simulink model "Practica_4"  (R2020b)
settings: Solver=VariableStepAuto  StartTime=0.0  StopTime=inf  RelTol=1e-3
model workspace (MAT data in the model file):
  alpha = Simulink.Parameter
  alpha.Value = 0.04
  alpha.DataType = 'auto'
  alpha.Dimensions = [1 1]
  dt = Simulink.Parameter
  dt.Value = 0.01
  dt.DataType = 'auto'
  dt.Dimensions = [1 1]
undefined symbols (not defined in the file or in its folder): serial
libraries: instrumentlib x2
settings Model: EnablePacing=on  Creator=eber_  LastModifiedBy=eber_

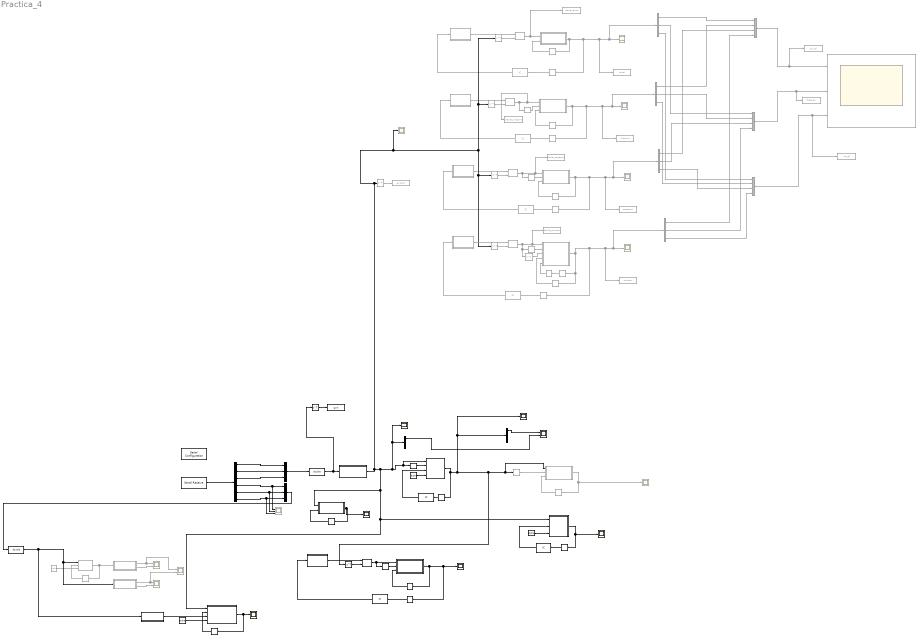
== system Practica_4 ==
  #nofilter : Scope  Commented=on  NumInputPorts=2
  #nofilter1 : Scope  Commented=on  NumInputPorts=2
  Chart : Stateflow chart  TreatAsAtomicUnit=on
  Data Type Conversion : DataTypeConversion  OutDataTypeStr=double
  Data Type Conversion2 : DataTypeConversion  OutDataTypeStr=double
  Delay : Delay  Commented=on
  Demux{,1..3} (4 alike) : Demux  Commented=on  Outputs=3
  Demux4 : Demux  Outputs=6
  Demux6 : Demux  Outputs=3
  Demux7 : Demux  Outputs=3
  Eul Angles{,2..4} (4 alike) : Scope  Commented=on
  Eul Angles1 : Scope
  Euler : MATLAB Function  Commented=on  TreatAsAtomicUnit=on
  Euler1 : MATLAB Function  TreatAsAtomicUnit=on
  Gyro1 : Scope  Commented=on
  IC{,2..4} (4 alike) : InitialCondition  Commented=on  Value=[0; 0; 0]
  IC1 : InitialCondition  Value=[0, 0, 0]
  IC5 : InitialCondition  Value=[0, 0, 0]
  IC6 : InitialCondition  Value=[0; 0; 0]
  MATLAB Function : MATLAB Function  Commented=on  TreatAsAtomicUnit=on
  MATLAB Function1 : MATLAB Function  Commented=on  TreatAsAtomicUnit=on
  MATLAB Function2 : MATLAB Function  Commented=on  TreatAsAtomicUnit=on
  MATLAB Function3 : MATLAB Function  TreatAsAtomicUnit=on
  MATLAB Function4 : MATLAB Function  TreatAsAtomicUnit=on
  MATLAB Function5 : MATLAB Function  TreatAsAtomicUnit=on
  MATLAB Function6 : MATLAB Function  TreatAsAtomicUnit=on
  Matrix Multiply{,1..3} (4 alike) : Product  Commented=on  Multiplication=Matrix(*)
  Matrix Multiply4 : Product  Multiplication=Matrix(*)
  Memory{,1..8,10..11,15} (12 alike) : Memory  Commented=on
  Memory12 : Memory  Commented=on  InheritSampleTime=on
  Memory13 : Memory  Commented=on  InheritSampleTime=on
  Memory14 : Memory  Commented=on  InitialCondition=[0, 0, 0]
  Memory{16,18..23} (7 alike) : Memory
  Memory17 : Memory  InitialCondition=[0, 0, 0]
  Memory9 : Memory  Commented=on  InheritSampleTime=on
  Midpoint : MATLAB Function  Commented=on  TreatAsAtomicUnit=on
  Mux : Mux  Commented=on
  Mux1 : Mux  Commented=on
  Mux2 : Mux  Commented=on
  Mux3 : Mux  Inputs=3
  Mux4 : Mux  Inputs=3
  Scope : Scope  Commented=on  NumInputPorts=3
  Scope1 : Scope  Commented=on
  Scope2 : Scope  Commented=on  NumInputPorts=3
  Scope{3..4,6..8} (5 alike) : Scope
  Scope5 : Scope  NumInputPorts=2
  Serial Configuration : instrumentlib/Serial Configuration  Priority=-200000  ComPortMenu=<Please select a port...>  ComPort=COM3  ObjConstructor=serial('COM3');  BaudRate=115200  DataBits=8  Parity=none  StopBits=1  FlowControl=none  Timeout=10  ByteOrder=LittleEndian
  Serial Receive : instrumentlib/Serial Receive  ComPortMenu=<Please select a port...>  ComPort=COM3  ObjConstructor=serial('COM3');  Terminator=<none>  DataSize="[1  6]"  DataType=single  EnableBlockingMode=on  ActionDataUnavailable=Output last received value  CustomValue=0  SampleTime=0.02
  Simpson : MATLAB Function  Commented=on  TreatAsAtomicUnit=on
  To Workspace1 : ToWorkspace  Commented=on  VariableName=euler  SaveFormat=Structure With Time  SampleTime=-1
  To Workspace10 : ToWorkspace  Commented=on  VariableName=deuler_simpson  SaveFormat=Structure With Time  SampleTime=-1
  To Workspace11 : ToWorkspace  Commented=on  VariableName=psi_all  SaveFormat=Structure With Time  SampleTime=-1
  To Workspace12 : ToWorkspace  Commented=on  VariableName=theta_all  SaveFormat=Structure With Time  SampleTime=-1
  To Workspace13 : ToWorkspace  Commented=on  VariableName=phi_all  SaveFormat=Structure With Time  SampleTime=-1
  To Workspace2 : ToWorkspace  VariableName=gyro  SaveFormat=Structure With Time  SampleTime=-1
  To Workspace3 : ToWorkspace  Commented=on  VariableName=gyrocorr  SaveFormat=Structure With Time  SampleTime=-1
  To Workspace4 : ToWorkspace  Commented=on  VariableName=midpoint  SaveFormat=Structure With Time  SampleTime=-1
  To Workspace5 : ToWorkspace  Commented=on  VariableName=trapezoid  SaveFormat=Structure With Time  SampleTime=-1
  To Workspace6 : ToWorkspace  Commented=on  VariableName=simpson  SaveFormat=Structure With Time  SampleTime=-1
  To Workspace7 : ToWorkspace  Commented=on  VariableName=deuler_euler  SaveFormat=Structure With Time  SampleTime=-1
  To Workspace8 : ToWorkspace  Commented=on  VariableName=deuler_midpoint  SaveFormat=Structure With Time  SampleTime=-1
  To Workspace9 : ToWorkspace  Commented=on  VariableName=deuler_trapezoid  SaveFormat=Structure With Time  SampleTime=-1
  Transformation Matrix : MATLAB Function  Commented=on  TreatAsAtomicUnit=on
  Transformation Matrix1 : MATLAB Function  Commented=on  TreatAsAtomicUnit=on
  Transformation Matrix2 : MATLAB Function  Commented=on  TreatAsAtomicUnit=on
  Transformation Matrix3 : MATLAB Function  Commented=on  TreatAsAtomicUnit=on
  Transformation Matrix4 : MATLAB Function  TreatAsAtomicUnit=on
  Transpose{,1..3,5} (5 alike) : Math  Commented=on  Operator=transpose  SaturateOnIntegerOverflow=on
  Transpose4 : Math  Operator=transpose  SaturateOnIntegerOverflow=on
  Transpose6 : Math  Operator=transpose  SaturateOnIntegerOverflow=on
  Trapezoid : MATLAB Function  Commented=on  TreatAsAtomicUnit=on
  Trapezoid1 : MATLAB Function  Commented=on  TreatAsAtomicUnit=on
  Trapezoid2 : MATLAB Function  TreatAsAtomicUnit=on
  alpha : Constant  Commented=on  Value=alpha
  alpha1 : Constant  Value=alpha
  alpha2 : Constant  Value=alpha
  alpha3 : Constant  Value=alpha
  filtered : Scope  Commented=on  NumInputPorts=2
  wires:
  Data Type Conversion/1 -> Transpose4/1, Chart/1(gyroIn)
  Euler/1(Euler_out) -> Memory/1, Memory1/1, To Workspace1/1, Eul Angles/1, Demux3/1
  IC/1 -> Transformation Matrix/1(Phi)
  Memory1/1 -> IC/1
  Memory/1 -> Euler/2(Euler)
  Transformation Matrix/1(H) -> Matrix Multiply/1
  Transpose/1 -> Matrix Multiply/2
  Matrix Multiply/1 -> To Workspace7/1, Euler/1(Euler_dot)
  Matrix Multiply1/1 -> Memory4/1, To Workspace8/1, Midpoint/1(Euler_dot)
  Transpose1/1 -> Matrix Multiply1/2
  Transformation Matrix1/1(H) -> Matrix Multiply1/1
  Memory3/1 -> Midpoint/3(Euler)
  Memory5/1 -> IC2/1
  IC2/1 -> Transformation Matrix1/1(Phi)
  Midpoint/1(Euler_out) -> Demux2/1, Eul Angles2/1, To Workspace4/1, Memory5/1, Memory3/1
  Memory4/1 -> Midpoint/2(Euler_dot_prev)
  Memory7/1 -> Trapezoid/2(Euler_dot_prev)
  Trapezoid/1(Euler_out) -> Memory6/1, Memory8/1, To Workspace5/1, Demux/1, Eul Angles3/1
  IC3/1 -> Transformation Matrix2/1(Phi)
  Memory8/1 -> IC3/1
  Memory6/1 -> Trapezoid/3(Euler)
  Transformation Matrix2/1(H) -> Matrix Multiply2/1
  Transpose2/1 -> Matrix Multiply2/2
  Matrix Multiply2/1 -> To Workspace9/1, Trapezoid/1(Euler_dot), Memory7/1
  Matrix Multiply3/1 -> Delay/1, Memory10/1, To Workspace10/1, Simpson/1(Euler_dot)
  Chart/1(gyroOut) -> MATLAB Function5/1(G), MATLAB Function4/1(G), Euler1/1(Euler_dot), Scope4/1, Demux7/1, Memory17/1, MATLAB Function3/1(U), Transpose/1, Transpose1/1, Transpose3/1, Transpose2/1, Gyro1/1, Transpose5/1  "raw"
  Transpose3/1 -> Matrix Multiply3/2
  Transformation Matrix3/1(H) -> Matrix Multiply3/1
  Memory9/1 -> Simpson/4(Euler_prev)
  Memory11/1 -> IC4/1
  IC4/1 -> Transformation Matrix3/1(Phi)
  Simpson/1(Euler_out) -> Memory9/1, Memory13/1, Demux1/1, Eul Angles4/1, To Workspace6/1, Memory11/1
  Memory10/1 -> Simpson/2(Euler_dot_prev)
  Memory12/1 -> Simpson/5(Euler_prev2)
  Delay/1 -> Simpson/3(Euler_dot_prev2)
  Demux3/1 -> Mux/1
  Demux2/1 -> Mux/2
  Demux/1 -> Mux/3
  Demux1/1 -> Mux/4
  Demux3/2 -> Mux1/1
  Demux2/2 -> Mux1/2
  Demux/2 -> Mux1/3
  Demux1/2 -> Mux1/4
  Demux3/3 -> Mux2/1
  Demux2/3 -> Mux2/2
  Demux/3 -> Mux2/3
  Demux1/3 -> Mux2/4
  Mux/1 -> To Workspace13/1, Scope/1
  Mux1/1 -> To Workspace12/1, Scope/2
  Mux2/1 -> To Workspace11/1, Scope/3
  Memory13/1 -> Memory12/1
  Transpose5/1 -> To Workspace3/1
  Transpose4/1 -> To Workspace2/1
  Serial Receive/1 -> Demux4/1
  Demux4/2 -> Mux3/2
  Demux4/1 -> Mux3/1
  Demux4/3 -> Mux3/3
  Demux4/5 -> Scope2/2, Mux4/2
  Demux4/4 -> Scope2/1, Mux4/1
  Demux4/6 -> Scope2/3, Mux4/3
  Mux3/1 -> Data Type Conversion/1  "gyro"
  Mux4/1 -> Data Type Conversion2/1  "acc"
  MATLAB Function1/1(X) -> MATLAB Function/1(acc), Memory2/1
  MATLAB Function/1(phi_acc) -> #nofilter1/1, filtered/1
  MATLAB Function/2(theta_acc) -> filtered/2
  Memory2/1 -> MATLAB Function1/2(Xa)
  alpha/1 -> MATLAB Function1/3(alpha)
  MATLAB Function2/2(theta_acc) -> #nofilter/2
  Data Type Conversion2/1 -> MATLAB Function2/1(acc), MATLAB Function1/1(U), MATLAB Function6/1(acc)
  MATLAB Function2/1(phi_acc) -> #nofilter1/2, #nofilter/1
  Memory14/1 -> Trapezoid1/3(Euler)
  Trapezoid1/1(Euler_out) -> Memory14/1, Scope1/1
  Memory15/1 -> Trapezoid1/2(Euler_dot_prev)
  Memory16/1 -> IC1/1
  alpha1/1 -> MATLAB Function3/4(alpha)
  Memory17/1 -> MATLAB Function3/2(Ua)
  IC1/1 -> MATLAB Function3/3(Xa)
  Demux6/1 -> Scope5/1
  Demux7/1 -> Scope5/2
  Memory18/1 -> Euler1/2(Euler)
  Euler1/1(Euler_out) -> Scope6/1, Memory18/1
  Memory19/1 -> IC5/1
  MATLAB Function4/1(X) -> Scope7/1, Memory19/1
  IC5/1 -> MATLAB Function4/2(Xa)
  alpha2/1 -> MATLAB Function4/3(alpha)
  IC6/1 -> Transformation Matrix4/1(Phi)
  Trapezoid2/1(Euler_out) -> Memory20/1, Memory22/1, Eul Angles1/1
  MATLAB Function3/1(X) -> Transpose6/1, Memory15/1, Trapezoid1/1(Euler_dot), Demux6/1, Scope3/1, Memory16/1  "raw"
  Memory21/1 -> Trapezoid2/2(Euler_dot_prev)
  Memory22/1 -> IC6/1
  Matrix Multiply4/1 -> Trapezoid2/1(Euler_dot), Memory21/1
  Transpose6/1 -> Matrix Multiply4/2
  Transformation Matrix4/1(H) -> Matrix Multiply4/1
  Memory20/1 -> Trapezoid2/3(Euler)
  Memory23/1 -> MATLAB Function5/2(Xa)
  MATLAB Function5/1(X) -> Scope8/1, Memory23/1
  MATLAB Function6/1(angAcc) -> MATLAB Function5/3(angAcc)
  alpha3/1 -> MATLAB Function5/4(alpha)

== matlab function Practica_4/Transformation Matrix3 ==
  data: Phi input; H output
function H = fcn(Phi)
Phi = deg2rad(Phi);

phi = Phi(1);
theta = Phi(2);
psi = Phi(3);

H = [1 tan(theta)*sin(phi) tan(theta)*cos(phi);
    0 cos(phi) -sin(phi);
    0 sin(phi)/cos(theta) cos(phi)/cos(theta)];

== matlab function Practica_4/Simpson ==
  data: Euler_dot input; Euler_dot_prev input; Euler_dot_prev2 input; Euler_out output; Euler_prev input; Euler_prev2 input
function Euler_out = fcn(Euler_dot, Euler_dot_prev, Euler_dot_prev2, Euler_prev, Euler_prev2)
dt = 0.02;

phi_dot = Euler_dot(1);
theta_dot = Euler_dot(2);
psi_dot = Euler_dot(3);

phi_dot_prev = Euler_dot_prev(1);
theta_dot_prev = Euler_dot_prev(2);
psi_dot_prev = Euler_dot_prev(3);

phi_dot_prev2 = Euler_dot_prev2(1);
theta_dot_prev2 = Euler_dot_prev2(2);
psi_dot_prev2 = Euler_dot_prev2(3);

phi_prev = Euler_prev(1);
theta_prev = Euler_prev(2);
psi_prev = Euler_prev(3);

phi_prev2 = Euler_prev2(1);
theta_prev2 = Euler_prev2(2);
psi_prev2 = Euler_prev2(3);

phi = phi_prev2 + (dt/3)*(phi_dot_prev2 + 4*phi_dot_prev + phi_dot);
theta = theta_prev2 + (dt/3)*(theta_dot_prev2 + 4*theta_dot_prev + theta_dot);
psi = psi_prev2 + (dt/3)*(psi_dot_prev2 + 4*psi_dot_prev + psi_dot);

Euler_out = [phi; theta; psi];

== matlab function Practica_4/MATLAB Function1 ==
  data: U input; X output; Xa input; alpha input
function X = fcn(U, Xa, alpha)
X = alpha*U + (1 - alpha)*Xa;

== matlab function Practica_4/MATLAB Function2 ==
  data: acc input; phi_acc output; theta_acc output
function [phi_acc, theta_acc] = fcn(acc)
ax = acc(1);
ay = acc(2);
az = acc(3);

phi_acc = atand(ax/sqrt(ay^2 + az^2));
theta_acc = atand(ay/sqrt(ax^2 + az^2));

== matlab function Practica_4/Trapezoid1 ==
  data: Euler_dot input; Euler_dot_prev input; Euler_out output; Euler input
function Euler_out = fcn(Euler_dot, Euler_dot_prev, Euler)
dt = 0.02;

phi_dot = Euler_dot(1);
theta_dot = Euler_dot(2);
psi_dot = Euler_dot(3);


phi_dot_prev = Euler_dot_prev(1);
theta_dot_prev = Euler_dot_prev(2);
psi_dot_prev = Euler_dot_prev(3);


phi = Euler(1);
theta = Euler(2);
psi = Euler(3);


phi = phi + dt*phi_dot - dt*((phi_dot - phi_dot_prev)/2);
theta = theta + dt*theta_dot - dt*((theta_dot - theta_dot_prev)/2);
psi = psi + dt*psi_dot - dt*((psi_dot - psi_dot_prev)/2);

Euler_out = [phi; theta; psi];

== matlab function Practica_4/MATLAB Function3 ==
  data: U input size=[1 3]; Ua input size=[1 3]; Xa input size=[1 3]; X output size=[1 3]; alpha input
function X = fcn(U, Ua, Xa, alpha)
X = Xa*(1- alpha) + (U - Ua);

== matlab function Practica_4/Euler1 ==
  data: Euler_dot input size=[1 3]; Euler_out output size=[1 3]; Euler input size=[1 3]
function Euler_out = fcn(Euler_dot, Euler)
dt = 0.02;
phi_dot = Euler_dot(1);
theta_dot = Euler_dot(2);
psi_dot = Euler_dot(3);

phi = Euler(1);
theta = Euler(2);
psi = Euler(3);


phi = phi + dt*phi_dot;
theta = theta + dt*theta_dot;
psi = psi + dt*psi_dot;

Euler_out = [phi, theta, psi];

== matlab function Practica_4/MATLAB Function4 ==
  data: G input size=[1 3]; Xa input size=[1 3]; X output size=[1 3]; alpha input
function X = fcn(G, Xa, alpha)
dt = 0.02;
X = Xa*(1 - alpha) + G*dt;

== matlab function Practica_4/Transformation Matrix4 ==
  data: Phi input; H output
function H = fcn(Phi)
Phi = deg2rad(Phi);

phi = Phi(1);
theta = Phi(2);
psi = Phi(3);

H = [1 tan(theta)*sin(phi) tan(theta)*cos(phi);
    0 cos(phi) -sin(phi);
    0 sin(phi)/cos(theta) cos(phi)/cos(theta)];

== matlab function Practica_4/Trapezoid2 ==
  data: Euler_dot input; Euler_dot_prev input; Euler_out output; Euler input
function Euler_out = fcn(Euler_dot, Euler_dot_prev, Euler)
dt = 0.02;

phi_dot = Euler_dot(1);
theta_dot = Euler_dot(2);
psi_dot = Euler_dot(3);


phi_dot_prev = Euler_dot_prev(1);
theta_dot_prev = Euler_dot_prev(2);
psi_dot_prev = Euler_dot_prev(3);


phi = Euler(1);
theta = Euler(2);
psi = Euler(3);


phi = phi + dt*phi_dot - dt*((phi_dot - phi_dot_prev)/2);
theta = theta + dt*theta_dot - dt*((theta_dot - theta_dot_prev)/2);
psi = psi + dt*psi_dot - dt*((psi_dot - psi_dot_prev)/2);

Euler_out = [phi; theta; psi];

== matlab function Practica_4/MATLAB Function5 ==
  data: G input; X output; Xa input; angAcc input; alpha input
function X = fcn(G, Xa, angAcc, alpha)
dt = 0.02;
G = [G(1), -G(2), G(3)]
X = (1 - alpha)*(Xa + G*dt) + alpha*angAcc;

== matlab function Practica_4/MATLAB Function6 ==
  data: acc input; angAcc output
function angAcc  = fcn(acc)
ax = acc(1);
ay = acc(2);
az = acc(3);

phi_acc = atand(ax/sqrt(ay^2 + az^2));
theta_acc = atand(ay/sqrt(ax^2 + az^2));
psi_acc = 0;

angAcc = [theta_acc, phi_acc, psi_acc]

== matlab function Practica_4/Euler ==
  data: Euler_dot input; Euler_out output; Euler input
function Euler_out = fcn(Euler_dot, Euler)
dt = 0.02;
phi_dot = Euler_dot(1);
theta_dot = Euler_dot(2);
psi_dot = Euler_dot(3);

phi = Euler(1);
theta = Euler(2);
psi = Euler(3);


phi = phi + dt*phi_dot;
theta = theta + dt*theta_dot;
psi = psi + dt*psi_dot;

Euler_out = [phi; theta; psi];

== matlab function Practica_4/Transformation Matrix ==
  data: Phi input; H output
function H = fcn(Phi)
Phi = deg2rad(Phi);

phi = Phi(1);
theta = Phi(2);
psi = Phi(3);

H = [1 tan(theta)*sin(phi) tan(theta)*cos(phi);
    0 cos(phi) -sin(phi);
    0 sin(phi)/cos(theta) cos(phi)/cos(theta)];

== matlab function Practica_4/MATLAB Function ==
  data: acc input; phi_acc output; theta_acc output
function [phi_acc, theta_acc] = fcn(acc)
ax = acc(1);
ay = acc(2);
az = acc(3);

phi_acc = atand(ax/sqrt(ay^2 + az^2));
theta_acc = atand(ay/sqrt(ax^2 + az^2));

== matlab function Practica_4/Midpoint ==
  data: Euler_dot input; Euler_dot_prev input; Euler_out output; Euler input
function Euler_out = fcn(Euler_dot, Euler_dot_prev, Euler)
dt = 0.02;

phi_dot = Euler_dot(1);
theta_dot = Euler_dot(2);
psi_dot = Euler_dot(3);


phi_dot_prev = Euler_dot_prev(1);
theta_dot_prev = Euler_dot_prev(2);
psi_dot_prev = Euler_dot_prev(3);


phi = Euler(1);
theta = Euler(2);
psi = Euler(3);


phi = phi + dt*((phi_dot + phi_dot_prev)/2);
theta = theta + dt*((theta_dot + theta_dot_prev)/2);
psi = psi + dt*((psi_dot + psi_dot_prev)/2);

Euler_out = [phi; theta; psi];

== matlab function Practica_4/Transformation Matrix1 ==
  data: Phi input; H output
function H = fcn(Phi)
Phi = deg2rad(Phi);

phi = Phi(1);
theta = Phi(2);
psi = Phi(3);

H = [1 tan(theta)*sin(phi) tan(theta)*cos(phi);
    0 cos(phi) -sin(phi);
    0 sin(phi)/cos(theta) cos(phi)/cos(theta)];

== stateflow chart Practica_4/Chart ==
  state initialSample
    entry:
    gyroOut = [0, 0, 0];
    pSum = 0;
    qSum = 0;
    rSum = 0;
    counter = 0;
    during:
    p = gyroIn(1);
    q = gyroIn(2);
    r = gyroIn(3);
    counter = counter + 1;
    pSum = pSum + p;
    qSum = qSum + q;
    rSum = rSum + r;
  state average
    entry:
    pOffset = pSum/counter;
    qOffset = qSum/counter;
    rOffset = rSum/counter;
    exit:
    offsets = [pOffset; qOffset; rOffset];
  state dataAcquisition
    during:
    p = gyroIn(1);
    q = gyroIn(2);
    r = gyroIn(3);
    pcorr = p - pOffset;
    qcorr = q - qOffset;
    rcorr = r - rOffset;
    gyroOut = [pcorr, qcorr, rcorr];
  (default) -> initialSample
  initialSample -> average : after(10, sec)
  average -> dataAcquisition
  data: counter local; p local; pOffset local; pSum local; r local; rOffset local; rSum local; q local; qOffset local; qSum local; offsets local; gyroOut output; pcorr local; qcorr local; rcorr local; gyroIn input

== matlab function Practica_4/Trapezoid ==
  data: Euler_dot input; Euler_dot_prev input; Euler_out output; Euler input
function Euler_out = fcn(Euler_dot, Euler_dot_prev, Euler)
dt = 0.02;

phi_dot = Euler_dot(1);
theta_dot = Euler_dot(2);
psi_dot = Euler_dot(3);


phi_dot_prev = Euler_dot_prev(1);
theta_dot_prev = Euler_dot_prev(2);
psi_dot_prev = Euler_dot_prev(3);


phi = Euler(1);
theta = Euler(2);
psi = Euler(3);


phi = phi + dt*phi_dot - dt*((phi_dot - phi_dot_prev)/2);
theta = theta + dt*theta_dot - dt*((theta_dot - theta_dot_prev)/2);
psi = psi + dt*psi_dot - dt*((psi_dot - psi_dot_prev)/2);

Euler_out = [phi; theta; psi];

== matlab function Practica_4/Transformation Matrix2 ==
  data: Phi input; H output
function H = fcn(Phi)
Phi = deg2rad(Phi);

phi = Phi(1);
theta = Phi(2);
psi = Phi(3);

H = [1 tan(theta)*sin(phi) tan(theta)*cos(phi);
    0 cos(phi) -sin(phi);
    0 sin(phi)/cos(theta) cos(phi)/cos(theta)];
